simulink model "Sim_YZ"  (R2016a)
settings: Solver=VariableStepAuto  StartTime=0.0  StopTime=10.0  RelTol=1e-3
values from neighbouring files (symbols this model uses):
  A_yz = double(subs(A_yz_temp,[x_yz u_yz],[0 0 0 0 0]))    [Systemdesign_YZ.m]
  B_yz = double(subs(B_yz_temp,[x_yz u_yz],[0 0 0 0 0]))    [Systemdesign_YZ.m]
  C_yz = eye(4)    [Systemdesign_YZ.m]
undefined symbols (not defined in the file or in its folder): K_yz
settings Model: Creator=Florian  LastModifiedBy=Florian

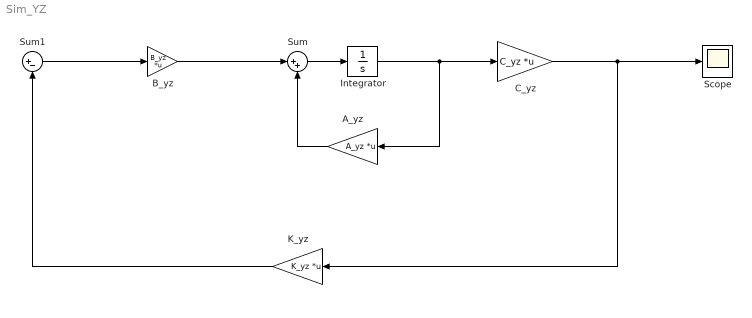
== system Sim_YZ ==
  A_yz : Gain  Gain=A_yz  Multiplication=Matrix(K*u) (u vector)
  B_yz : Gain  Gain=B_yz  Multiplication=Matrix(K*u)
  "C_yz " : Gain  Gain=C_yz  Multiplication=Matrix(K*u) (u vector)
  Integrator : Integrator
  "K_yz " : Gain  Gain=K_yz  Multiplication=Matrix(K*u) (u vector)
  Scope : Scope
  Sum : Sum  Inputs=|++
  Sum1 : Sum  Inputs=|+-
  wires:
  A_yz/1 -> Sum/2
  Sum/1 -> Integrator/1
  Integrator/1 -> A_yz/1, "C_yz "/1
  "C_yz "/1 -> Scope/1, "K_yz "/1
  B_yz/1 -> Sum/1
  "K_yz "/1 -> Sum1/2
  Sum1/1 -> B_yz/1
